simulink model "PID_SISO"  (R2025b)
settings: Solver=VariableStepAuto  StartTime=0.0  StopTime=10.0  RelTol=1e-3
libraries: Drone_SISO_Subsystem x1
settings Model: Creator=Alek  LastModifiedBy=Alek
settings DataIOCC: ExternalInput=getinputstruct(report2)  InitialState=getstatestruct(report2)  LoadExternalInput=on  LoadInitialState=on

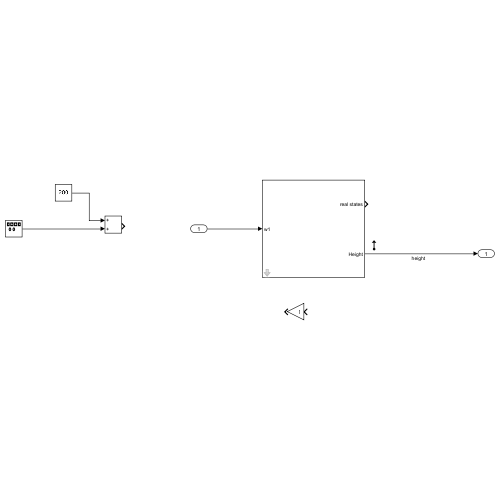
[thumbnail: Simulink's stored preview of the top-level diagram]
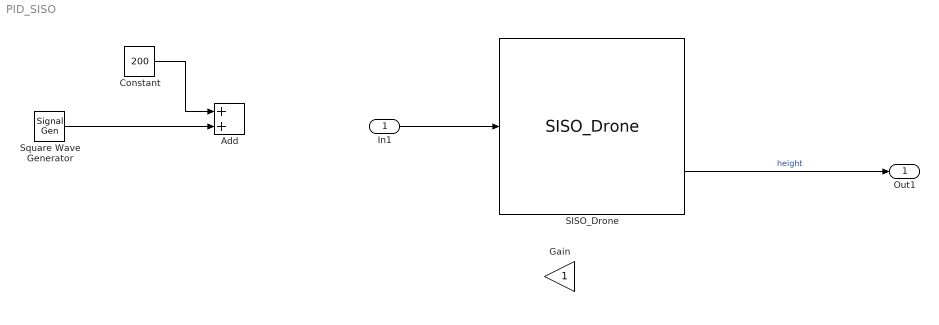
== system PID_SISO ==
  In1 : Inport
  Add : Sum
  Constant : Constant  Value=200
  Gain : Gain
  SISO_Drone : Drone_SISO_Subsystem/SISO_Drone  kf=1e-5  m=0.5  l=1e-2  I=6.6666e-5
      settings: SourceProductName=Drone SISO Plant
  Square Wave Generator : SignalGenerator  WaveForm=square  Frequency=0.1  Units=rad/sec
  Out1 : Outport
  wires:
  Constant/1 -> Add/1
  Square Wave Generator/1 -> Add/2
  SISO_Drone/2 -> Out1/1  "height"
  In1/1 -> SISO_Drone/1
